simulink model "pump_3"  (R2018a)
settings: Solver=VariableStepDiscrete  StartTime=0.0  StopTime=3  RelTol=1e-3
values from neighbouring files (symbols this model uses):
  Ts = 0.0001    [pump_ori_perf.mat]
libraries: fl_lib x8, sh_lib x5, nesl_utility x5, powerlib x3, powerlib_meascontrol x2, electricdrivelib x1
settings Model: Creator=siwak  LastModifiedBy=siwak

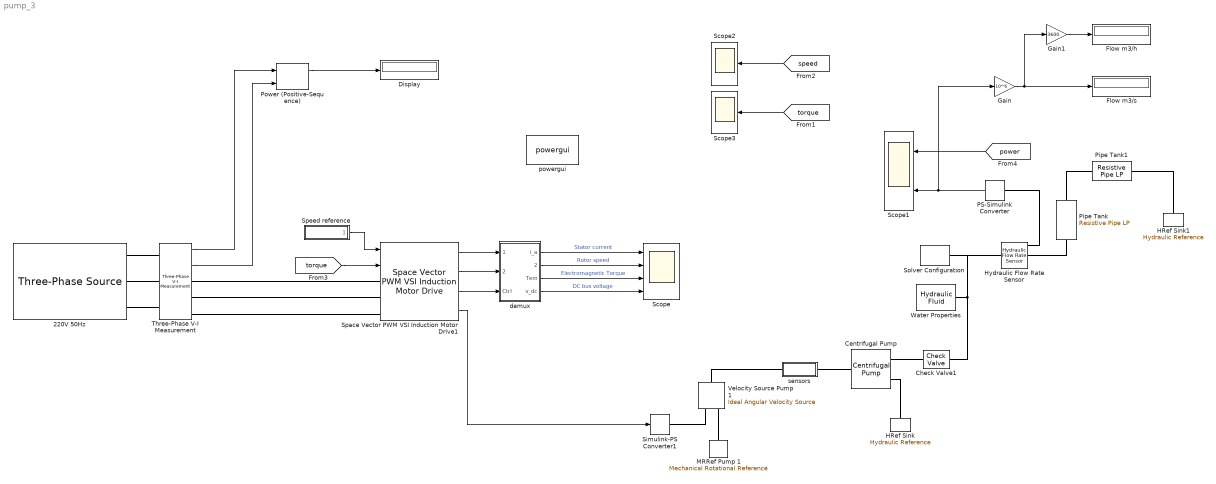
== system pump_3 ==
  220V 50Hz : powerlib/Electrical Sources/Three-Phase Source  InternalConnection=Yg  VoltagePhases=off  Voltage=220  PhaseAngle=0  Voltage_phases=[25e3 25e3 25e3]/sqrt(3)  PhaseAngles_phases=[0 -120 +120]  Frequency=50  NonIdealSource=on  SpecifyImpedance=off  Resistance=0.02  Inductance=0.05e-3  ShortCircuitLevel=100e6  BaseVoltage=25e3  XRratio=7  BusType=swing  Pref=0  Qref=0  Prefabc=[10e3, 10e3, 10e3]  Qrefabc=[0, 0, 0]  Qmin=-inf  Qmax=inf
  Centrifugal Pump : sh_lib/Pumps and Motors/Centrifugal Pump  mdl_type=2  c_1=326.8 Pa/(kg/m^3)  c_2=3.104e+4 Pa*s/kg  c_3=1.097e+7 Pa*s^2/(kg*m^3)  c_4=2.136e+5 Pa*s^2/(kg*m^3)  c_f=0.8  design_del=130 lpm  ref_velocity=1800 rpm  ref_density=940 kg/m^3  leak_resistance=1e+8 Pa/(m^3/s)  T_const=0.1 N*m  trq_press_coeff=1e-6 N*m/Pa  pump_del_1D="[0    1.8927    6.0756    8.7822   10.4099   12.3026] gpm"  press_diff_1D="[1274.3         1177          978       784.75          590       392.25] psi"  pump_del_power_1D="[0         500        1605        2320        2750        3250] gpm"  power_1D="[0          3.9         10.5           12         10.8          8.5] HP"  pump_vel_2D=[ 3.2e+3 3.3e+3 3.4e+3 3.5e+3 ] rpm  pump_del_2D=[ 0 50 100 150 200 250 300 350 ] lpm  press_diff_2D=[ 8.3 8.8 9.3 9.9; 7.8 8.3 8.8 9.4; 7.2 7.6 8.2 8.7; 6.5 7 7.5 8; 5.6 6.1 6.6 7.1; 4.7 5.2 5.7 6.2; 3.4 4 4.4 4.9; 2.3 2.7 3.4 3.6 ] bar  pump_del_power_2D=[ 0 50 100 150 200 250 300 350 ] lpm  power_2D=[ 1.223e+3 1.341e+3 1.467e+3 1.6e+3; 1.414e+3 1.551e+3 1.696e+3 1.85e+3; 1.636e+3 1.794e+3 1.962e+3 2.14e+3; 1.941e+3 2.129e+3 2.326e+3 2.54e+3; 2.224e+3 2.439e+3 2.66e+3 2.91e+3; 2.453e+3 2.691e+3 2.947e+3 3.21e+3; 2.757e+3 3.024e+3 3.307e+3 3.608e+3; 2.945e+3 3.23e+3 3.533e+3 3.854e+3 ] W  omega_threshold=1e-9 rad/s  interp_method=1  extrap_method=1
      settings: SourceProductName=Simscape Fluids  SourceProductBaseCode=SH
  Check Valve1 : sh_lib/Valves/Directional Valves/Check Valve  area_max=3.8 in^2  pres_crack=0.8 psi  pres_max=2.5 psi  C_d=0.7  A_leak=1e-9 m^2  lam_spec=1  B_lam=0.999  Re_cr=12  dynamic=0  tau=0.1 s  area_init=1e-12 m^2
      settings: SourceProductName=Simscape Fluids  SourceProductBaseCode=SH
  Display : Display
  Flow m3/h : Display
      settings: Decimation=2
  Flow m3/s : Display
      settings: Decimation=2
  Gain : Gain  Gain=10^6
  Gain1 : Gain  Gain=3600
  HRef Sink : fl_lib/Hydraulic/Hydraulic Elements/Hydraulic Reference
      settings: SourceProductName=Simscape
  HRef Sink1 : fl_lib/Hydraulic/Hydraulic Elements/Hydraulic Reference
      settings: SourceProductName=Simscape
  Hydraulic Flow Rate Sensor : fl_lib/Hydraulic/Hydraulic Sensors/Hydraulic Flow Rate Sensor
      settings: SourceProductName=Simscape
  MRRef Pump 1 : fl_lib/Mechanical/Rotational Elements/Mechanical Rotational Reference
  PS-Simulink Converter : nesl_utility/PS-Simulink Converter  PhysicalDomain=network_engine_domain  SubClassName=ps_output  LeftPortType=input  RightPortType=output  PseudoPeriodic=off  Frequencies=[]  Unit=m^3/s  AffineConversion=off
  Pipe Tank : sh_lib/Low-Pressure Blocks/Resistive Pipe LP  cs_type=1  d_in=10 in  area=1e-4 m^2  D_h=0.0112 m  s_factor=64  length=1.5 m  length_ad=1 m  roughness=1.5e-5 m  Re_lam=2e+3  Re_turb=4e+3  elevation_A=0.5 m  elevation_B=2 m  g=9.80665 m/s^2  pressure_drop_specify=off  pressure_drop_priority=None  pressure_drop=0 Pa  pressure_drop_nominal_specify=off  pressure_drop_nominal_unit=Pa  pressure_drop_nominal_value=1  flow_rate_specify=off  flow_rate_priority=None  flow_rate=0 m^3/s  flow_rate_nominal_specify=off  flow_rate_nominal_unit=m^3/s  flow_rate_nominal_value=1
      settings: SourceProductName=Simscape Fluids  SourceProductBaseCode=SH
  Pipe Tank1 : sh_lib/Low-Pressure Blocks/Resistive Pipe LP  cs_type=1  d_in=10 in  area=1e-4 m^2  D_h=0.0112 m  s_factor=64  length=5 m  length_ad=1 m  roughness=1.5e-5 m  Re_lam=2e+3  Re_turb=4e+3  elevation_A=2 m  elevation_B=2 m  g=9.80665 m/s^2  pressure_drop_specify=off  pressure_drop_priority=None  pressure_drop=0 Pa  pressure_drop_nominal_specify=off  pressure_drop_nominal_unit=Pa  pressure_drop_nominal_value=1  flow_rate_specify=off  flow_rate_priority=None  flow_rate=0 m^3/s  flow_rate_nominal_specify=off  flow_rate_nominal_unit=m^3/s  flow_rate_nominal_value=1
      settings: SourceProductName=Simscape Fluids  SourceProductBaseCode=SH
  Power (Positive-Sequence) : powerlib_meascontrol/Measurements/Power (Positive-Sequence)  Freq=60  Vinit=[220 0]  Iinit=[0 0]  Ts=Ts
      settings: SourceProductName=Simscape Power Systems  SourceProductBaseCode=PS
  Scope : Scope  NumInputPorts=4
  Scope1 : Scope  NumInputPorts=2
  Scope2 : Scope
  Scope3 : Scope
  Simulink-PS Converter1 : nesl_utility/Simulink-PS Converter  PhysicalDomain=network_engine_domain  SubClassName=ps_input  LeftPortType=input  RightPortType=output  PseudoPeriodic=off  Frequencies=[]  NoiseDistribution=none  NoiseParameters=[]  Unit=rpm  AffineConversion=off  FilteringAndDerivatives=zero  SimscapeFilterOrder=1  InputFilterTimeConstant=.001  UdotUserProvided=0
  Solver Configuration : nesl_utility/Solver Configuration  PhysicalDomain=network_engine_domain  SubClassName=solver  LeftPortType=input  RightPortType=generic  Tones=[]  Harmonics=[]  SimulateNoise=off  Profile=off  UseLocalSampling=off  EnableSwitchedLinearOptims=on  FrequencyDomain=off  UseCCode=off  RelTol=0.001  AbsTol=1e-06  MinStep=1e-09  ToWorkspace=off  RevertToSquareIcSolve=off  NumHomotopyIterations=100  PhasorMode=off  PhasorModeNumHarmonics=1  DoDC=off  ResidualTolerance=1e-9  UseLocalSolver=on  LocalSolverChoice=NE_BACKWARD_EULER_ADVANCER  LocalSolverSampleTime=.001  DoFixedCost=on  MaxNonlinIter=3  MaxModeIter=2  LinearAlgebra=Sparse  EquationFormulation=NE_TIME_EF  DelaysMemoryBudget=1024  AutomaticFiltering=on  FilteringTimeConstant=0.001
  Space Vector PWM VSI Induction Motor Drive1 : electricdrivelib/AC drives/Space Vector PWM VSI Induction Motor Drive  ReferenceFrame=Stationary  IterativeDiscreteModel=Trapezoidal non iterative  Pn=50000  Vn=220  fn=50  Rs=0.435  Lls=0.002  Lms=69.31e-3  Rr=0.816  Llr=0.002  ia=0  pha=0  ib=0  phb=0  ic=0  phc=0  J=0.140  Friction=0.005  p=4  slip=1  thdeg=0  Rsnb_rec=10e3  Csnb_rec=20e-9  Ron_rec=1e-3  Vf_rec=1.3  cap_bus=3400e-6  Rbrake=8  fbrake=4000  activationVoltage=340  shutdownVoltage=320  deviceType=IGBT / Diodes  Ron_inv=1e-3  Vf_inv=1.2  Vfd_inv=1.2  Tf=1e-6  Tt=2e-6  Tf_GTO=10e-6  Tt_GTO=20e-6  Rsnb_inv=500  Csnb_inv=1e-9  Acc=1800  Dec=-1800  kp_sc=9  ki_sc=10  fc_sc=100  Tsc=100e-6  ctrl_sat_min=-30  ctrl_sat_max=30  ctrl_f_min=0.05  ctrl_f_max=120  ctrl_v_min=10  ctrl_v_max=180  vh_ratio=3.2  zc_time=0.4  car_freq=4500  fc_bus=50  Tvect=20e-6  baseSampleTime=2e-06  outputBusMode=Multiple output buses  busLabels=off  MechanicalLoad=Torque Tm  modelDetailLevel=Detailed  driveType=AC2  AverageValue=off
      settings: SourceProductName=Simscape Power Systems  SourceProductBaseCode=PS
  Speed reference : Subsystem
  Three-Phase V-I Measurement : powerlib/Measurements/Three-Phase V-I Measurement  VoltageMeasurement=phase-to-ground  SetLabelV=off  LabelV=Vabc  Vpu=off  VpuLL=off  CurrentMeasurement=yes  SetLabelI=off  LabelI=Iabc  Ipu=off  Pbase=100e6  Vbase=500e3  OutputType=Complex  PhasorSimulation=off  PSBequivalent=0
  Velocity Source Pump 1 : fl_lib/Mechanical/Mechanical Sources/Ideal Angular Velocity Source
  Water Properties : sh_lib/Hydraulic Utilities/Hydraulic Fluid  DataSource=1  SelFluid=24  SysTemp=1  TrapAir=0.001  ViscDerFactor=1  range_error=2
      settings: SourceProductName=Simscape Fluids
  demux : Subsystem
  powergui : powerlib/powergui  Priority=2  SimulationMode=Discrete  SampleTime=Ts  frequency=60  Iterations=50  frequencyindice=50  Pbase=100e6  ErrMax=1e-4  UnitsV=kV  UnitsW=MW  buscounter=0  FunctionMessages=off  echomessages=off  EnableUseOfTLC=off  CurrentSourceSwitches=off  DisableSnubberDevices=off  DisableRonSwitches=off  DisableVfSwitches=off  DisplayEquations=off  SolverType=Tustin/Backward Euler (TBE)  Interpol=off  ExternalGateDelay=off  methode=off  Ts=100  x0status=blocks  SPID=off  SwTol=0  HookPort=off  RestoreLinks=warning  ResistiveCurrentMeasurement=off  Frange=[0:2:500]  Ylog=off  Xlog=on  ShowGrid=off  save=off  variable=ZData  structure=0  ZoomFFT=on  StartTime=0.0  cycles=1  DisplayStyle=1  fundamental=60  FreqAxis=off  MaxFrequency=1000  frequencyindicesteady=1  RmsSteady=1  display=off
  sensors : Subsystem
  wires:
  demux/3(Tem) -> Scope/3  "Electromagnetic Torque"
  Space Vector PWM VSI Induction Motor Drive1/2 -> demux/2(Conv.)
  Space Vector PWM VSI Induction Motor Drive1/3 -> demux/3(Ctrl)
  Space Vector PWM VSI Induction Motor Drive1/4 -> Simulink-PS Converter1/1
  Speed reference/1(" ") -> Space Vector PWM VSI Induction Motor Drive1/1
  Space Vector PWM VSI Induction Motor Drive1/1 -> demux/1(Motor)
  demux/2(speed) -> Scope/2  "Rotor speed"
  demux/4(v_dc) -> Scope/4  "DC bus voltage"
  demux/1(i_a) -> Scope/1  "Stator current"
  [torque] -> Space Vector PWM VSI Induction Motor Drive1/2
  [speed] -> Scope2/1
  [torque] -> Scope3/1
  PS-Simulink Converter/1 -> Gain/1, Scope1/2
  [power] -> Scope1/1
  Three-Phase V-I Measurement/2 -> Power (Positive-Sequence)/2
  Three-Phase V-I Measurement/1 -> Power (Positive-Sequence)/1
  Power (Positive-Sequence)/1 -> Display/1
  Gain/1 -> Gain1/1, Flow m3/s/1
  Gain1/1 -> Flow m3/h/1
  connections:
  Simulink-PS Converter1/RConn1 -- Velocity Source Pump 1/RConn1
  MRRef Pump 1/LConn1 -- Velocity Source Pump 1/RConn2
  sensors/LConn1 -- Velocity Source Pump 1/LConn1
  Centrifugal Pump/LConn1 -- sensors/RConn1
  Centrifugal Pump/RConn2 -- HRef Sink/LConn1
  Solver Configuration/RConn1 -- Hydraulic Flow Rate Sensor/LConn1 -- Check Valve1/RConn1 -- Water Properties/RConn1
  Pipe Tank/LConn1 -- Hydraulic Flow Rate Sensor/RConn2
  Pipe Tank1/LConn1 -- Pipe Tank/RConn1
  Hydraulic Flow Rate Sensor/RConn1 -- PS-Simulink Converter/LConn1
  Check Valve1/LConn1 -- Centrifugal Pump/RConn1
  Pipe Tank1/RConn1 -- HRef Sink1/LConn1
  Three-Phase V-I Measurement/LConn1 -- 220V 50Hz/RConn1
  Three-Phase V-I Measurement/LConn2 -- 220V 50Hz/RConn2
  Three-Phase V-I Measurement/LConn3 -- 220V 50Hz/RConn3
  Space Vector PWM VSI Induction Motor Drive1/LConn1 -- Three-Phase V-I Measurement/RConn1
  Space Vector PWM VSI Induction Motor Drive1/LConn2 -- Three-Phase V-I Measurement/RConn2
  Space Vector PWM VSI Induction Motor Drive1/LConn3 -- Three-Phase V-I Measurement/RConn3

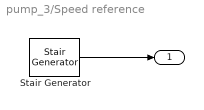
== system pump_3/Speed reference ==
  Stair Generator : powerlib_meascontrol/Pulse & Signal Generators/Stair Generator  t=[0.1]  e=[1800]  Ts=Ts
      settings: SourceProductName=Simscape Power Systems
  " " : Outport
  wires:
  Stair Generator/1 -> " "/1

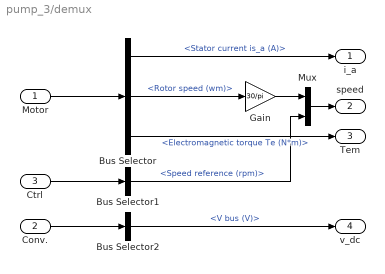
== system pump_3/demux ==
  Motor : Inport
  Conv. : Inport  Port=2
  Ctrl : Inport  Port=3
  Bus Selector : BusSelector  OutputSignals=Stator measurements.Stator current is_a (A),Mechanical.Rotor speed (wm),Mechanical.Electromagnetic torque Te (N*m)
  Bus Selector1 : BusSelector  OutputSignals=Speed reference (rpm)
  Bus Selector2 : BusSelector  OutputSignals=V bus (V)
  Gain : Gain  Gain=30/pi  SaturateOnIntegerOverflow=on  OutDataTypeStr=Inherit: Same as input  ParamDataTypeStr=Inherit: Same as input
  Mux : Mux  Inputs=2
  i_a : Outport
  speed : Outport  Port=2
  Tem : Outport  Port=3
  v_dc : Outport  Port=4
  wires:
  Ctrl/1 -> Bus Selector1/1
  Gain/1 -> Mux/1
  Mux/1 -> speed/1
  Motor/1 -> Bus Selector/1
  Bus Selector/1 -> i_a/1  "<Stator current is_a (A)>"
  Bus Selector/2 -> Gain/1  "<Rotor speed (wm)>"
  Bus Selector/3 -> Tem/1  "<Electromagnetic torque Te (N*m)>"
  Bus Selector1/1 -> Mux/2  "<Speed reference (rpm)>"
  Conv./1 -> Bus Selector2/1
  Bus Selector2/1 -> v_dc/1  "<V bus (V)>"

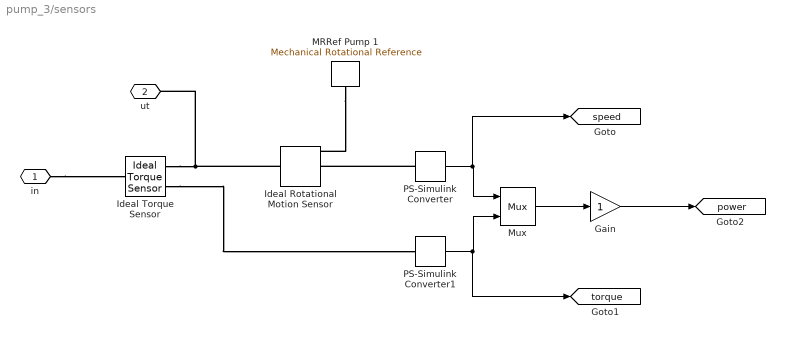
== system pump_3/sensors ==
  Gain : Gain
  Ideal Rotational Motion Sensor : fl_lib/Mechanical/Mechanical Sensors/Ideal Rotational Motion Sensor  offset=0 rad
  Ideal Torque Sensor : fl_lib/Mechanical/Mechanical Sensors/Ideal Torque Sensor
  MRRef Pump 1 : fl_lib/Mechanical/Rotational Elements/Mechanical Rotational Reference
  Mux : Mux  Inputs=2
  PS-Simulink Converter : nesl_utility/PS-Simulink Converter  PhysicalDomain=network_engine_domain  SubClassName=ps_output  LeftPortType=input  RightPortType=output  PseudoPeriodic=off  Frequencies=[]  Unit=rad/s  AffineConversion=off
  PS-Simulink Converter1 : nesl_utility/PS-Simulink Converter  PhysicalDomain=network_engine_domain  SubClassName=ps_output  LeftPortType=input  RightPortType=output  PseudoPeriodic=off  Frequencies=[]  Unit=N*m  AffineConversion=off
  in : PMIOPort  Side=Left
  ut : PMIOPort  Port=2  Side=Right
  tag scope: power=global, speed=global, torque=global
  wires:
  PS-Simulink Converter/1 -> [speed], Mux/1
  PS-Simulink Converter1/1 -> [torque], Mux/2
  Mux/1 -> Gain/1
  Gain/1 -> [power]
  connections:
  in/RConn1 -- Ideal Torque Sensor/LConn1
  Ideal Torque Sensor/RConn1 -- Ideal Rotational Motion Sensor/LConn1 -- ut/RConn1
  MRRef Pump 1/LConn1 -- Ideal Rotational Motion Sensor/RConn1
  PS-Simulink Converter/LConn1 -- Ideal Rotational Motion Sensor/RConn2
  Ideal Torque Sensor/RConn2 -- PS-Simulink Converter1/LConn1
